simulink model "sih_top_model"  (R2026a)
settings: Solver=FixedStepDiscrete  FixedStep=0.1
InitFcn:
  | sihDefineBuses();
values from neighbouring files (symbols this model uses):
  egoStub = Simulink.Bus.createMATLABStruct('SihEgoBus')    [sihBuildTopModel.m]
  perceptionStub = Simulink.Bus.createMATLABStruct('SihPerceptionBus')    [sihBuildTopModel.m]
settings Model: Creator=ROSHAN KUMAR C  LastModifiedBy=ROSHAN KUMAR C

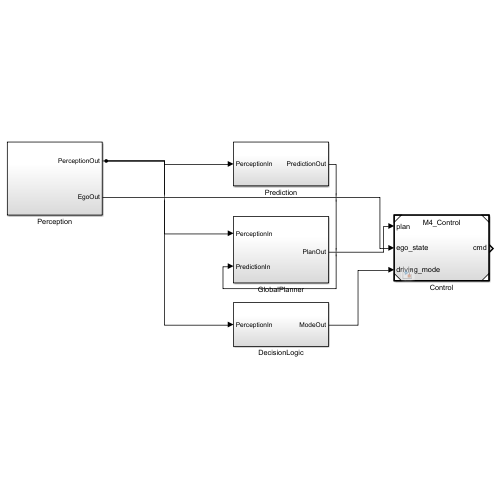
[thumbnail: Simulink's stored preview of the top-level diagram]
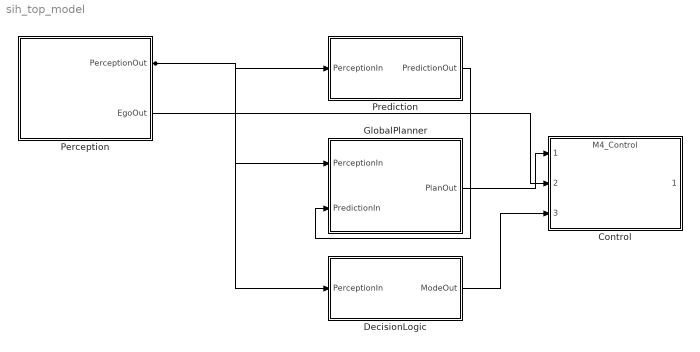
== system sih_top_model ==
  Control : ModelReference  ModelNameDialog=M4_Control  SimulationMode=Normal  ModelReferenceVersion=1.3
  DecisionLogic : Subsystem
  GlobalPlanner : Subsystem
  Perception : Subsystem
  Prediction : Subsystem
  wires:
  Perception/1(PerceptionOut) -> Prediction/1(PerceptionIn), GlobalPlanner/1(PerceptionIn), DecisionLogic/1(PerceptionIn)
  Prediction/1(PredictionOut) -> GlobalPlanner/2(PredictionIn)
  GlobalPlanner/1(PlanOut) -> Control/1
  Perception/2(EgoOut) -> Control/2
  DecisionLogic/1(ModeOut) -> Control/3

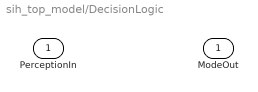
== system sih_top_model/DecisionLogic ==
  PerceptionIn : Inport
  ModeOut : Outport
  wires:
  ? -> ?

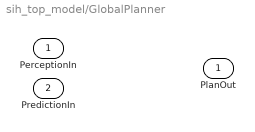
== system sih_top_model/GlobalPlanner ==
  PerceptionIn : Inport
  PredictionIn : Inport  Port=2
  PlanOut : Outport
  wires:
  ? -> ?

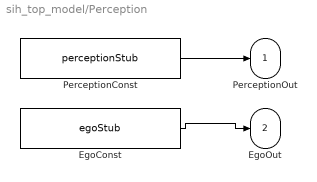
== system sih_top_model/Perception ==
  EgoConst : Constant  Value=egoStub
  PerceptionConst : Constant  Value=perceptionStub
  PerceptionOut : Outport
  EgoOut : Outport  Port=2
  wires:
  ? -> ?
  PerceptionConst/1 -> PerceptionOut/1
  EgoConst/1 -> EgoOut/1

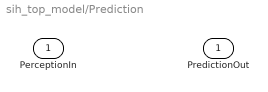
== system sih_top_model/Prediction ==
  PerceptionIn : Inport
  PredictionOut : Outport
  wires:
  ? -> ?
